simulink model "ObserverBased_Controller"  (R2020b)
settings: Solver=VariableStepAuto  StartTime=0.0  StopTime=10.0  RelTol=1e-3
libraries: pid_lib x1
settings Model: Creator=Kevin  LastModifiedBy=Kevin

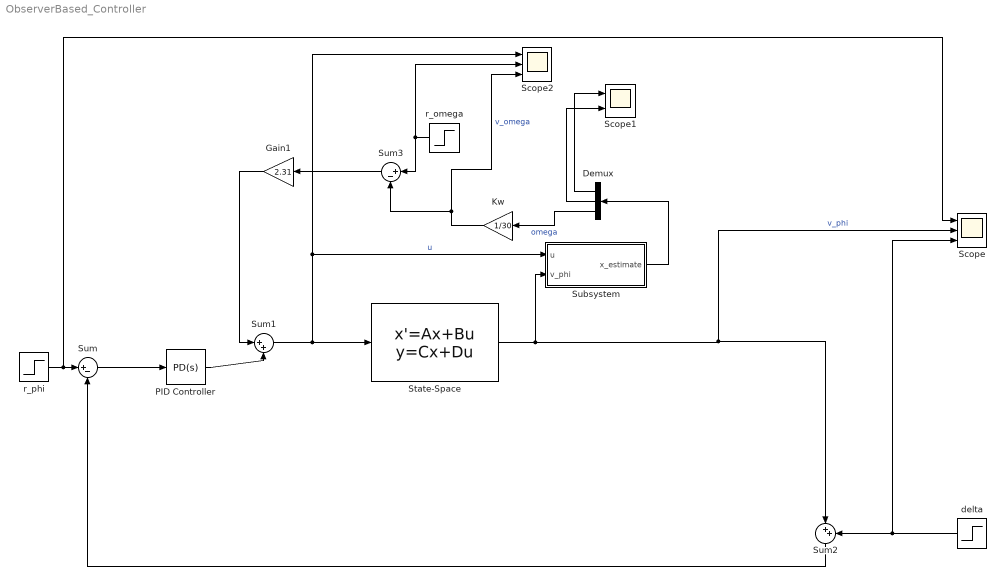
== system ObserverBased_Controller ==
  Demux : Demux  Outputs=3
  Gain1 : Gain  Gain=2.31
  Kw : Gain  Gain=1/30
  PID Controller : pid_lib/PID Controller  Controller=PD  Form=Ideal  TimeDomain=Continuous-time  UseExternalTs=off  SampleTime=-1  IntegratorMethod=Forward Euler  FilterMethod=Forward Euler  ControllerParametersSource=internal  P=21.3  I=1  D=0.21  UseFilter=on  N=100  TunerSelectOption=Transfer Function Based (PID Tuner App)  InitialConditionSource=internal  InitialConditionForIntegrator=0  InitialConditionForFilter=0  DifferentiatorICPrevScaledInput=0  ExternalReset=none  TrackingMode=off  Kt=1  LimitOutput=off  SatLimitsSource=internal  UpperSaturationLimit=inf  LowerSaturationLimit=-inf  LinearizeAsGain=on  AntiWindupMode=none  Kb=1  POutMin=[]  POutMax=[]  IOutMin=[]  IOutMax=[]  DOutMin=[]  DOutMax=[]  NOutMin=[]  NOutMax=[]  SumOutMin=[]  SumOutMax=[]  SaturationOutMin=[]  SaturationOutMax=[]  PParamMin=[]  PParamMax=[]  IParamMin=[]  IParamMax=[]  DParamMin=[]  DParamMax=[]  NParamMin=[]  NParamMax=[]  KbParamMin=[]  KbParamMax=[]  KtParamMin=[]  KtParamMax=[]  KbOutMin=[]  KbOutMax=[]  KtOutMin=[]  KtOutMax=[]  IntegratorOutMin=[]  IntegratorOutMax=[]  FilterOutMin=[]  FilterOutMax=[]  SumI1OutMin=[]  SumI1OutMax=[]  SumI2OutMin=[]  SumI2OutMax=[]  SumI3OutMin=[]  SumI3OutMax=[]  SumI4OutMin=[]  SumI4OutMax=[]  SumDOutMin=[]  SumDOutMax=[]  DifferentiatorOutMin=[]  DifferentiatorOutMax=[]  FilterDiffOutCoefMin=[]  FilterDiffOutCoefMax=[]  ReciprocalOutMin=[]  ReciprocalOutMax=[]  SumDenOutMin=[]  SumDenOutMax=[]  SumNumOutMin=[]  SumNumOutMax=[]  DivideOutMin=[]  DivideOutMax=[]  UdiffTsProdOutMin=[]  UdiffTsProdOutMax=[]  NTsProdOutMin=[]  NTsProdOutMax=[]  UintegralTsProdOutMin=[]  UintegralTsProdOutMax=[]  UngainTsProdOutMin=[]  UngainTsProdOutMax=[]  IntegratorContinuousStateAttributes=''  IntegratorStateMustResolveToSignalObject=off  IntegratorRTWStateStorageClass=Auto  FilterContinuousStateAttributes=''  FilterStateMustResolveToSignalObject=off  FilterRTWStateStorageClass=Auto  ParallelPVariant=Passthrough  IdealPVariant=InternalParameters  IVariant=Disabled  DVariant=InternalParameters  IntegratorVariant=Disabled  SatVariant=Disabled  AWVariant=Disabled  PCopyVariant=Disabled  TRVariant=Disabled  FdbkBlocksVariant=Forward  IdealPFdbkVariant=Disabled  SatFdbkVariant=Disabled  DerivativeFilterVariant=ContFilter  NVariant=InternalParameters  NCopyVariant=Disabled  FilterICVariant=InternalICsFilter  IntegratorICVariant=Disabled  ExternalResetVariant=Disabled  TRSumVariant=Passthrough  SumFdbkVariant=Disabled  SumVariant=Sum_PD  TsampFilterVariant=InternalTs  TsampNgainVariant=Passthrough  TsampIntegralVariant=Disabled_SignalSpec  ExternalSaturationOutDataTypeStr=Inherit: Same as second input
  Scope : Scope  NumInputPorts=3
  Scope1 : Scope  NumInputPorts=2
  Scope2 : Scope  NumInputPorts=3
  State-Space : StateSpace  A=[0 1 0; 23.5031 0 0.0045; -23.5031 0 -19.9513]  B=[0; 0.1393; -621.6819]  C=[107.47 0 0]  D=0  InitialCondition=[0.0019 0 0]
  Subsystem : Subsystem
  Sum : Sum  Inputs=|+-
  Sum1 : Sum  Inputs=|++
  Sum2 : Sum  Inputs=|++
  Sum3 : Sum  Inputs=|+-
  delta : Step  Time=1.5  After=0.2  SampleTime=0
  r_omega : Step  Time=2.5  After=2.5  SampleTime=0
  r_phi : Step  Time=0  After=0  SampleTime=0
  wires:
  r_phi/1 -> Scope/1, Sum/1
  Sum/1 -> PID Controller/1
  Gain1/1 -> Sum1/1
  PID Controller/1 -> Sum1/2
  Sum1/1 -> Scope2/1, Subsystem/1(u), State-Space/1  "u"
  State-Space/1 -> Subsystem/2(v_phi), Sum2/1, Scope/2  "v_phi"
  delta/1 -> Scope/3, Sum2/2
  Sum2/1 -> Sum/2
  Sum3/1 -> Gain1/1
  Subsystem/1(x_estimate) -> Demux/1
  Demux/3 -> Kw/1  "omega"
  Kw/1 -> Scope2/3, Sum3/2  "v_omega"
  r_omega/1 -> Scope2/2, Sum3/1
  Demux/1 -> Scope1/1
  Demux/2 -> Scope1/2

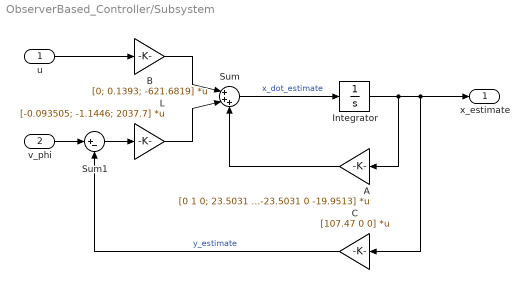
== system ObserverBased_Controller/Subsystem ==
  u : Inport
  v_phi : Inport  Port=2
  A : Gain  Gain=[0 1 0; 23.5031 0 0.0045; -23.5031 0 -19.9513]  Multiplication=Matrix(K*u)
  B : Gain  Gain=[0; 0.1393; -621.6819]  Multiplication=Matrix(K*u)
  C : Gain  Gain=[107.47 0 0]  Multiplication=Matrix(K*u)
  Integrator : Integrator
  L : Gain  Gain=[-0.093505; -1.1446; 2037.7]  Multiplication=Matrix(K*u)
  Sum : Sum  Inputs=|+++
  Sum1 : Sum  Inputs=|+-
  x_estimate : Outport
  wires:
  u/1 -> B/1
  v_phi/1 -> Sum1/1
  Sum1/1 -> L/1
  B/1 -> Sum/1
  Sum/1 -> Integrator/1  "x_dot_estimate"
  Integrator/1 -> A/1, C/1, x_estimate/1
  A/1 -> Sum/3
  C/1 -> Sum1/2  "y_estimate"
  L/1 -> Sum/2
